simulink model "DoubleIntQuad"  (R2021b)
settings: Solver=VariableStepAuto  StartTime=0.0  StopTime=100  RelTol=1e-3
values from neighbouring files (symbols this model uses):
  A = [0 1; 0 0]    [DoubleIntControllerDev.m]
  B = [0; 1/m]    [DoubleIntControllerDev.m]
  C = [1 0]    [DoubleIntControllerDev.m]
  K_lqi = lqi(sys,Q,R)    [DoubleIntControllerDev.m]
settings Model: Creator=renkert2  LastModifiedBy=renkert2

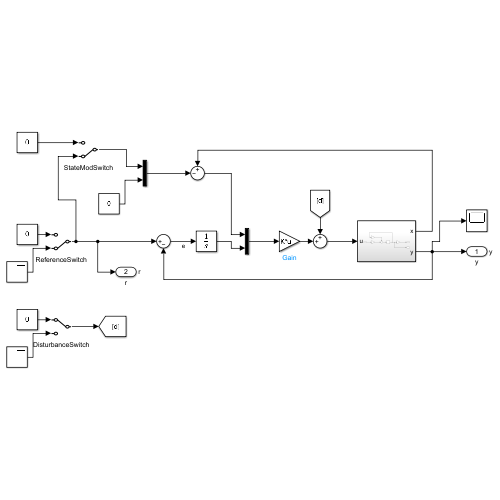
[thumbnail: Simulink's stored preview of the top-level diagram]
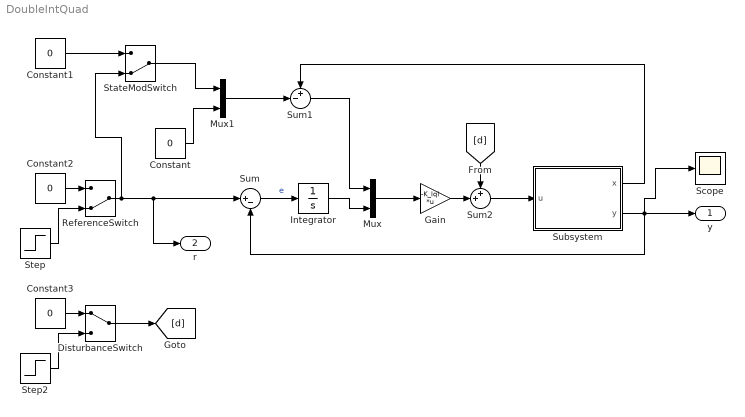
== system DoubleIntQuad ==
  Constant{,1..3} (4 alike) : Constant  Value=0
  DisturbanceSwitch : ManualSwitch
  Gain : Gain  Gain=-K_lqi  Multiplication=Matrix(K*u)
  Integrator : Integrator
  Mux : Mux  Inputs=2
  Mux1 : Mux  Inputs=2
  ReferenceSwitch : ManualSwitch  CurrentSetting=0
  Scope : Scope
  StateModSwitch : ManualSwitch  CurrentSetting=0
  Step : Step  SampleTime=0
  Step2 : Step  SampleTime=0
  Subsystem : Subsystem
  Sum : Sum  Inputs=|+-
  Sum1 : Sum  Inputs=+-|
  Sum2 : Sum  Inputs=++|
  y : Outport  SignalName=y
  r : Outport  Port=2  SignalName=r
  wires:
  Integrator/1 -> Mux/2
  Subsystem/2(y) -> Scope/1, y/1, Sum/2
  Sum/1 -> Integrator/1  "e"
  Mux/1 -> Gain/1
  Subsystem/1(x) -> Sum1/1
  Constant/1 -> Mux1/2
  Sum1/1 -> Mux/1
  Gain/1 -> Sum2/2
  Constant1/1 -> StateModSwitch/1
  StateModSwitch/1 -> Mux1/1
  Sum2/1 -> Subsystem/1(u)
  Constant2/1 -> ReferenceSwitch/1
  ReferenceSwitch/1 -> StateModSwitch/2, r/1, Sum/1
  Step/1 -> ReferenceSwitch/2
  Step2/1 -> DisturbanceSwitch/2
  Constant3/1 -> DisturbanceSwitch/1
  DisturbanceSwitch/1 -> [d]
  [d] -> Sum2/1
  Mux1/1 -> Sum1/2

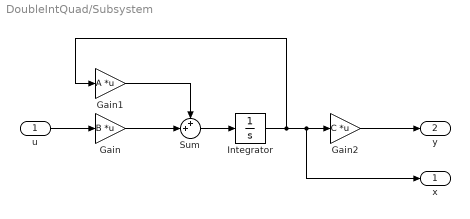
== system DoubleIntQuad/Subsystem ==
  u : Inport
  Gain : Gain  Gain=B  Multiplication=Matrix(K*u)
  Gain1 : Gain  Gain=A  Multiplication=Matrix(K*u)
  Gain2 : Gain  Gain=C  Multiplication=Matrix(K*u)
  Integrator : Integrator  InitialCondition=[0;0]
  Sum : Sum  Inputs=++|
  x : Outport
  y : Outport  Port=2
  wires:
  Gain/1 -> Sum/2
  Integrator/1 -> Gain1/1, x/1, Gain2/1
  Gain1/1 -> Sum/1
  Sum/1 -> Integrator/1
  u/1 -> Gain/1
  Gain2/1 -> y/1
